simulink model "bsm1_dyn_ASonly"  (R2012b)
settings: Solver=ode15s  SolverMode=SingleTasking  StartTime=0.0  StopTime=14  FixedStep=0.01  RelTol=1e-5  AbsTol=1e-8
values from neighbouring files (symbols this model uses):
  ACTIVATE = [ 0 ]    [init_bsm1.m]
  carb1 = 0    [reginit_bsm1.m]    (also in reginit_bsm1_2.m)
  carb2 = 0    [reginit_bsm1.m]    (also in reginit_bsm1_2.m)
  carb3 = 0    [reginit_bsm1.m]    (also in reginit_bsm1_2.m)
  carb4 = 0    [reginit_bsm1.m]    (also in reginit_bsm1_2.m)
  carb5 = 0    [reginit_bsm1.m]    (also in reginit_bsm1_2.m)
  KLa1 = 2    [reginit_bsm1.m]    (also in reginit_bsm1_2.m)
  KLa2 = 2    [reginit_bsm1.m]    (also in reginit_bsm1_2.m)
  KLa3 = 240    [reginit_bsm1.m]    (also in reginit_bsm1_2.m)
  KLa4 = 240    [reginit_bsm1.m]    (also in reginit_bsm1_2.m)
  KLa5 = 240    [reginit_bsm1.m]    (also in reginit_bsm1_2.m)
  PAR2 = PAR1    [mcsim.m]
  PAR3 = PAR1    [mcsim.m]
  PAR4 = PAR1    [mcsim.m]
  PAR5 = PAR1    [mcsim.m]
  TEMPMODEL = [ 0 ]    [init_bsm1.m]
undefined symbols (not defined in the file or in its folder): PAR1, SOSAT1, SOSAT2, SOSAT3, SOSAT4, SOSAT5, VOL1, VOL2, VOL3, VOL4, VOL5, XINIT1, XINIT2, XINIT3, XINIT4, XINIT5
settings Model: ExtModeTrigMode=oneshot  ExtModeArmWhenConnect=off  ExtModeAutoUpdateStatusClock=off  BufferReuse=off  Creator=ielulf  LastModifiedBy=lasn
settings DataIOCC: InitialState=xFinal  LimitDataPoints=off  SignalLoggingSaveFormat=ModelDataLogs  SaveOutput=off  TimeSaveName=t  SignalLoggingName=sigsOut  OutputOption=SpecifiedOutputTimes  OutputTimes=[0:(1/96):14]
settings OptimizationCC: BlockReduction=off  BooleanDataType=off  InlineInvariantSignals=on  OptimizeBlockIOStorage=off  BufferReuse=off  ExpressionFolding=off  LocalBlockOutputs=off  InitFltsAndDblsToZero=on
settings DebuggingCC: SaveWithParameterizedLinksMsg=none  SignalResolutionControl=TryResolveAllWithWarning  SolverPrmCheckMsg=none  InheritedTsInSrcMsg=none  MultiTaskDSMMsg=warning  MultiTaskCondExecSysMsg=none  FcnCallInpInsideContextMsg=UseLocalSettings  UnconnectedOutputMsg=none  StrictBusMsg=None
settings HardwareCC: TargetUnknown=on
settings RTWCC: TemplateMakefile=grt_unix.tmf  IncludeERTFirstTime=on
settings GRTTargetCC: TargetFcnLib=ansi_tfl_tmw.mat  CombineOutputUpdateFcns=off  GRTInterface=on

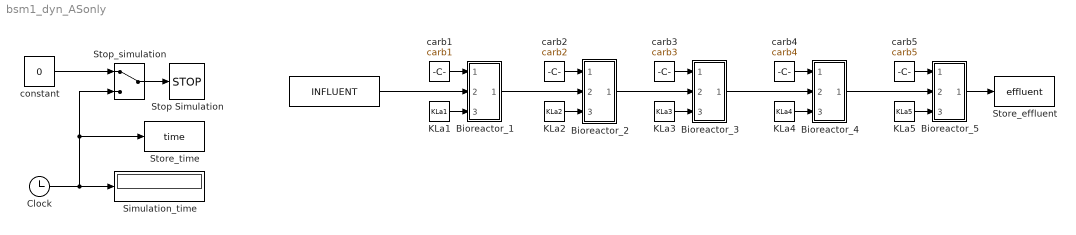
== system bsm1_dyn_ASonly ==
  " " : FromWorkspace  VariableName=INFLUENT  OutputAfterFinalValue=Holding final value
  " constant" : Constant  Value=0
  Bioreactor_1 : Subsystem
  Bioreactor_2 : Subsystem
  Bioreactor_3 : Subsystem
  Bioreactor_4 : Subsystem
  Bioreactor_5 : Subsystem
  Clock : Clock
  KLa1 : Constant  Value=KLa1
  KLa2 : Constant  Value=KLa2
  KLa3 : Constant  Value=KLa3
  KLa4 : Constant  Value=KLa4
  KLa5 : Constant  Value=KLa5
  Simulation_time : Display
  Stop Simulation : Stop
  Stop_simulation : ManualSwitch
  Store_effluent : ToWorkspace  VariableName=effluent
  Store_time : ToWorkspace  VariableName=time
  carb1 : Constant  Value=carb1
  carb2 : Constant  Value=carb2
  carb3 : Constant  Value=carb3
  carb4 : Constant  Value=carb4
  carb5 : Constant  Value=carb5
  wires:
  Clock/1 -> Simulation_time/1, Stop_simulation/2, Store_time/1
  Stop_simulation/1 -> Stop Simulation/1
  " constant"/1 -> Stop_simulation/1
  " "/1 -> Bioreactor_1/2(in)
  KLa1/1 -> Bioreactor_1/3(KLa)
  Bioreactor_1/1(out) -> Bioreactor_2/2(in)
  KLa2/1 -> Bioreactor_2/3(KLa)
  Bioreactor_2/1(out) -> Bioreactor_3/2(in)
  KLa3/1 -> Bioreactor_3/3(KLa)
  Bioreactor_3/1(out) -> Bioreactor_4/2(in)
  KLa4/1 -> Bioreactor_4/3(KLa)
  Bioreactor_4/1(out) -> Bioreactor_5/2(in)
  KLa5/1 -> Bioreactor_5/3(KLa)
  carb1/1 -> Bioreactor_1/1(carb)
  carb2/1 -> Bioreactor_2/1(carb)
  carb3/1 -> Bioreactor_3/1(carb)
  carb4/1 -> Bioreactor_4/1(carb)
  carb5/1 -> Bioreactor_5/1(carb)
  Bioreactor_5/1(out) -> Store_effluent/1

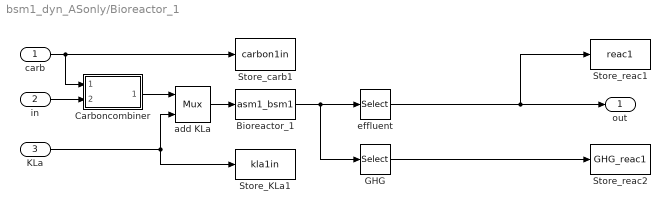
== system bsm1_dyn_ASonly/Bioreactor_1 ==
  carb : Inport
  in : Inport  Port=2
  KLa : Inport  Port=3
  Bioreactor_1 : S-Function  FunctionName=asm1_bsm1  Parameters=XINIT1,PAR1,VOL1,SOSAT1,TEMPMODEL,ACTIVATE  EnableBusSupport=off
  Carboncombiner : Subsystem
  GHG : Selector  InputPortWidth=29  IndexOptions=Index vector (dialog)  Indices=[27:29]  OutputSizes=1
  Store_KLa1 : ToWorkspace  VariableName=kla1in  SampleTime=-1
  Store_carb1 : ToWorkspace  VariableName=carbon1in  SampleTime=-1
  Store_reac1 : ToWorkspace  VariableName=reac1  SampleTime=-1
  Store_reac2 : ToWorkspace  VariableName=GHG_reac1  SampleTime=-1
  add KLa : Mux  Inputs=2
  effluent : Selector  InputPortWidth=29  IndexOptions=Index vector (dialog)  Indices=[1:26]  OutputSizes=1
  out : Outport
  wires:
  KLa/1 -> Store_KLa1/1, add KLa/2
  in/1 -> Carboncombiner/2(Input)
  carb/1 -> Carboncombiner/1(C_flow), Store_carb1/1
  Carboncombiner/1(Output) -> add KLa/1
  add KLa/1 -> Bioreactor_1/1
  Bioreactor_1/1 -> effluent/1, GHG/1
  effluent/1 -> out/1, Store_reac1/1
  GHG/1 -> Store_reac2/1

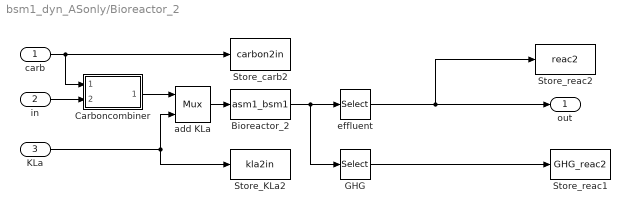
== system bsm1_dyn_ASonly/Bioreactor_2 ==
  carb : Inport
  in : Inport  Port=2
  KLa : Inport  Port=3
  Bioreactor_2 : S-Function  FunctionName=asm1_bsm1  Parameters=XINIT2,PAR2,VOL2,SOSAT2,TEMPMODEL,ACTIVATE  EnableBusSupport=off
  Carboncombiner : Subsystem
  GHG : Selector  InputPortWidth=29  IndexOptions=Index vector (dialog)  Indices=[27:29]  OutputSizes=1
  Store_KLa2 : ToWorkspace  VariableName=kla2in  SampleTime=-1
  Store_carb2 : ToWorkspace  VariableName=carbon2in  SampleTime=-1
  Store_reac1 : ToWorkspace  VariableName=GHG_reac2  SampleTime=-1
  Store_reac2 : ToWorkspace  VariableName=reac2  SampleTime=-1
  add KLa : Mux  Inputs=2
  effluent : Selector  InputPortWidth=29  IndexOptions=Index vector (dialog)  Indices=[1:26]  OutputSizes=1
  out : Outport
  wires:
  KLa/1 -> Store_KLa2/1, add KLa/2
  in/1 -> Carboncombiner/2(Input)
  carb/1 -> Store_carb2/1, Carboncombiner/1(C_flow)
  Carboncombiner/1(Output) -> add KLa/1
  add KLa/1 -> Bioreactor_2/1
  Bioreactor_2/1 -> GHG/1, effluent/1
  effluent/1 -> out/1, Store_reac2/1
  GHG/1 -> Store_reac1/1

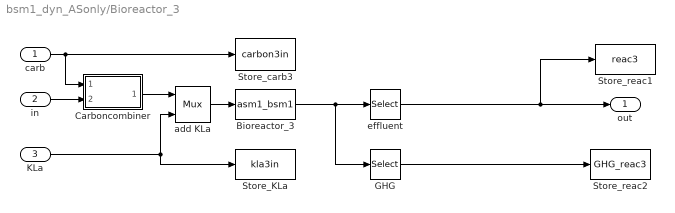
== system bsm1_dyn_ASonly/Bioreactor_3 ==
  carb : Inport
  in : Inport  Port=2
  KLa : Inport  Port=3
  Bioreactor_3 : S-Function  FunctionName=asm1_bsm1  Parameters=XINIT3,PAR3,VOL3,SOSAT3,TEMPMODEL,ACTIVATE  EnableBusSupport=off
  Carboncombiner : Subsystem
  GHG : Selector  InputPortWidth=29  IndexOptions=Index vector (dialog)  Indices=[27:29]  OutputSizes=1
  Store_KLa : ToWorkspace  VariableName=kla3in  SampleTime=-1
  Store_carb3 : ToWorkspace  VariableName=carbon3in  SampleTime=-1
  Store_reac1 : ToWorkspace  VariableName=reac3  SampleTime=-1
  Store_reac2 : ToWorkspace  VariableName=GHG_reac3  SampleTime=-1
  add KLa : Mux  Inputs=2
  effluent : Selector  InputPortWidth=29  IndexOptions=Index vector (dialog)  Indices=[1:26]  OutputSizes=1
  out : Outport
  wires:
  KLa/1 -> Store_KLa/1, add KLa/2
  in/1 -> Carboncombiner/2(Input)
  carb/1 -> Store_carb3/1, Carboncombiner/1(C_flow)
  Carboncombiner/1(Output) -> add KLa/1
  add KLa/1 -> Bioreactor_3/1
  Bioreactor_3/1 -> effluent/1, GHG/1
  effluent/1 -> out/1, Store_reac1/1
  GHG/1 -> Store_reac2/1

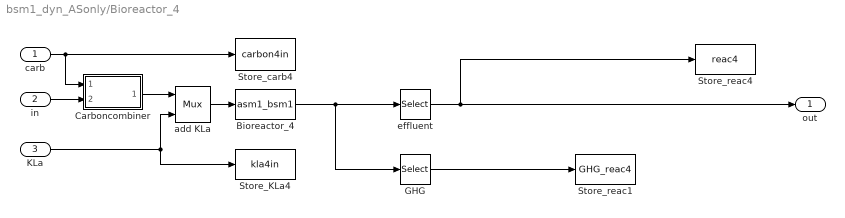
== system bsm1_dyn_ASonly/Bioreactor_4 ==
  carb : Inport
  in : Inport  Port=2
  KLa : Inport  Port=3
  Bioreactor_4 : S-Function  FunctionName=asm1_bsm1  Parameters=XINIT4,PAR4,VOL4,SOSAT4,TEMPMODEL,ACTIVATE  EnableBusSupport=off
  Carboncombiner : Subsystem
  GHG : Selector  InputPortWidth=29  IndexOptions=Index vector (dialog)  Indices=[27:29]  OutputSizes=1
  Store_KLa4 : ToWorkspace  VariableName=kla4in  SampleTime=-1
  Store_carb4 : ToWorkspace  VariableName=carbon4in  SampleTime=-1
  Store_reac1 : ToWorkspace  VariableName=GHG_reac4  SampleTime=-1
  Store_reac4 : ToWorkspace  VariableName=reac4  SampleTime=-1
  add KLa : Mux  Inputs=2
  effluent : Selector  InputPortWidth=29  IndexOptions=Index vector (dialog)  Indices=[1:26]  OutputSizes=1
  out : Outport
  wires:
  KLa/1 -> Store_KLa4/1, add KLa/2
  in/1 -> Carboncombiner/2(Input)
  carb/1 -> Store_carb4/1, Carboncombiner/1(C_flow)
  Carboncombiner/1(Output) -> add KLa/1
  add KLa/1 -> Bioreactor_4/1
  Bioreactor_4/1 -> GHG/1, effluent/1
  effluent/1 -> out/1, Store_reac4/1
  GHG/1 -> Store_reac1/1

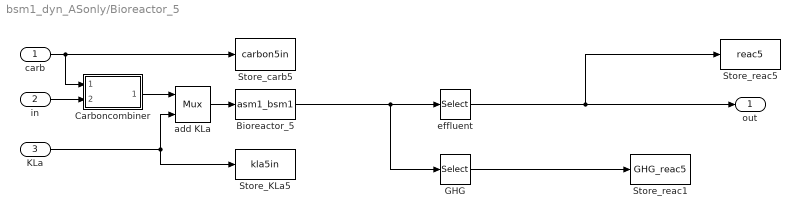
== system bsm1_dyn_ASonly/Bioreactor_5 ==
  carb : Inport
  in : Inport  Port=2
  KLa : Inport  Port=3
  Bioreactor_5 : S-Function  FunctionName=asm1_bsm1  Parameters=XINIT5,PAR5,VOL5,SOSAT5,TEMPMODEL,ACTIVATE  EnableBusSupport=off
  Carboncombiner : Subsystem
  GHG : Selector  InputPortWidth=29  IndexOptions=Index vector (dialog)  Indices=[27:29]  OutputSizes=1
  Store_KLa5 : ToWorkspace  VariableName=kla5in  SampleTime=-1
  Store_carb5 : ToWorkspace  VariableName=carbon5in  SampleTime=-1
  Store_reac1 : ToWorkspace  VariableName=GHG_reac5  SampleTime=-1
  Store_reac5 : ToWorkspace  VariableName=reac5  SampleTime=-1
  add KLa : Mux  Inputs=2
  effluent : Selector  InputPortWidth=29  IndexOptions=Index vector (dialog)  Indices=[1:26]  OutputSizes=1
  out : Outport
  wires:
  KLa/1 -> Store_KLa5/1, add KLa/2
  in/1 -> Carboncombiner/2(Input)
  carb/1 -> Store_carb5/1, Carboncombiner/1(C_flow)
  Carboncombiner/1(Output) -> add KLa/1
  add KLa/1 -> Bioreactor_5/1
  Bioreactor_5/1 -> GHG/1, effluent/1
  effluent/1 -> out/1, Store_reac5/1
  GHG/1 -> Store_reac1/1

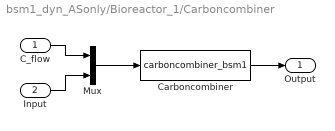
== system bsm1_dyn_ASonly/Bioreactor_1/Carboncombiner ==
  C_flow : Inport
  Input : Inport  Port=2
  Carboncombiner : S-Function  FunctionName=carboncombiner_bsm1  Parameters=CARBONSOURCECONC  EnableBusSupport=off
  Mux : Mux  Inputs=2
  Output : Outport
  wires:
  Input/1 -> Mux/2
  Carboncombiner/1 -> Output/1
  Mux/1 -> Carboncombiner/1
  C_flow/1 -> Mux/1

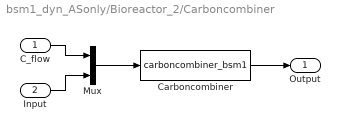
== system bsm1_dyn_ASonly/Bioreactor_2/Carboncombiner ==
  C_flow : Inport
  Input : Inport  Port=2
  Carboncombiner : S-Function  FunctionName=carboncombiner_bsm1  Parameters=CARBONSOURCECONC  EnableBusSupport=off
  Mux : Mux  Inputs=2
  Output : Outport
  wires:
  C_flow/1 -> Mux/1
  Mux/1 -> Carboncombiner/1
  Carboncombiner/1 -> Output/1
  Input/1 -> Mux/2

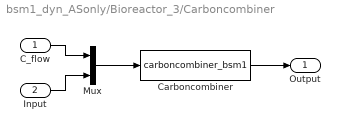
== system bsm1_dyn_ASonly/Bioreactor_3/Carboncombiner ==
  C_flow : Inport
  Input : Inport  Port=2
  Carboncombiner : S-Function  FunctionName=carboncombiner_bsm1  Parameters=CARBONSOURCECONC  EnableBusSupport=off
  Mux : Mux  Inputs=2
  Output : Outport
  wires:
  C_flow/1 -> Mux/1
  Mux/1 -> Carboncombiner/1
  Carboncombiner/1 -> Output/1
  Input/1 -> Mux/2

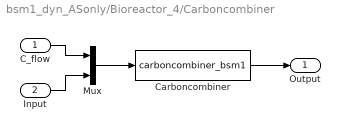
== system bsm1_dyn_ASonly/Bioreactor_4/Carboncombiner ==
  C_flow : Inport
  Input : Inport  Port=2
  Carboncombiner : S-Function  FunctionName=carboncombiner_bsm1  Parameters=CARBONSOURCECONC  EnableBusSupport=off
  Mux : Mux  Inputs=2
  Output : Outport
  wires:
  C_flow/1 -> Mux/1
  Mux/1 -> Carboncombiner/1
  Carboncombiner/1 -> Output/1
  Input/1 -> Mux/2

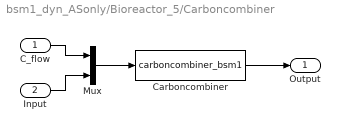
== system bsm1_dyn_ASonly/Bioreactor_5/Carboncombiner ==
  C_flow : Inport
  Input : Inport  Port=2
  Carboncombiner : S-Function  FunctionName=carboncombiner_bsm1  Parameters=CARBONSOURCECONC  EnableBusSupport=off
  Mux : Mux  Inputs=2
  Output : Outport
  wires:
  C_flow/1 -> Mux/1
  Mux/1 -> Carboncombiner/1
  Carboncombiner/1 -> Output/1
  Input/1 -> Mux/2
